simulink model "3_model"  (R2014b)
settings: Solver=ode45  StartTime=0.0  StopTime=10.0  RelTol=1e-3
settings Model: Creator=Shane Reynolds  LastModifiedBy=Shane Reynolds
settings DataIOCC: OutputSaveName=Output

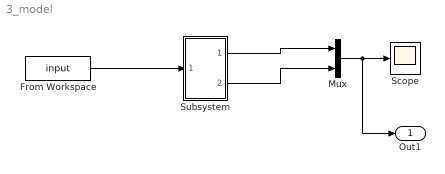
== system 3_model ==
  From Workspace : FromWorkspace  VariableName=input  SampleTime=0
  Mux : Mux  Inputs=2
  Scope : Scope
  Subsystem : Subsystem
  Out1 : Outport
  wires:
  Mux/1 -> Out1/1, Scope/1
  From Workspace/1 -> Subsystem/1(In1)
  Subsystem/1(Out1) -> Mux/1
  Subsystem/2(Out2) -> Mux/2

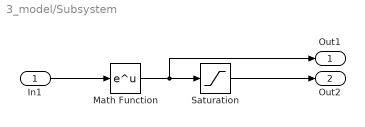
== system 3_model/Subsystem ==
  In1 : Inport
  Math Function : Math  SaturateOnIntegerOverflow=on
  Saturation : Saturate  UpperLimit=2  LowerLimit=0.5
  Out1 : Outport
  Out2 : Outport  Port=2
  wires:
  In1/1 -> Math Function/1
  Saturation/1 -> Out2/1
  Math Function/1 -> Out1/1, Saturation/1
